simulink model "salirClaseStateFlow"  (R2021b)
settings: Solver=FixedStepAuto  StartTime=0.0  StopTime=inf  RelTol=1e-3  EnableMultiTasking=on
StartFcn:
  | dg = 0.2
model workspace (MAT data in the model file):
  dg = 0.2
settings Model: ExtModeTrigDuration=2  Creator=Mauri  LastModifiedBy=Mauri
settings OptimizationCC: EnhancedBackFolding=on  PassReuseOutputArgsAs=Individual arguments  ZeroExternalMemoryAtStartup=off  ZeroInternalMemoryAtStartup=off  MaxStackSize=64  OptimizeBlockOrder=speed  DifferentSizesBufferReuse=on  OptimizationCustomize=off  EfficientTunableParamExpr=on
settings DebuggingCC: ParameterTunabilityLossMsg=error
settings HardwareCC: ProdBitPerInt=16  ProdBitPerPointer=16  ProdBitPerSizeT=16  ProdBitPerPtrDiffT=16  ProdLargestAtomicFloat=None  ProdWordSize=8  ProdHWDeviceType=Atmel->AVR  UseEmbeddedCoderFeatures=off  UseSimulinkCoderFeatures=off
settings SFSimCC: MATLABDynamicMemAlloc=off
settings RTWCC: Description=Embedded Coder  SystemTargetFile=ert.tlc  HardwareBoard=Arduino Mega 2560  TemplateMakefile=ert_default_tmf  Toolchain=Arduino AVR  BuildConfiguration=Faster Runs
settings CodeAppCC: ForceParamTrailComments=on  IgnoreCustomStorageClasses=off  OperatorAnnotations=on  SimulinkDataObjDesc=on  SFDataObjDesc=on  InsertBlockDesc=on
settings ERTTargetCC: SupportContinuousTime=on  SupportNonInlinedSFcns=on  SupportVariableSizeSignals=on  ExtModeTransport=3  ExtModeStaticAlloc=on  ExtModeStaticAllocSize=2048  ExtModeMexFile=ext_xcp  ExtModeIntrfLevel=Level2 - Open

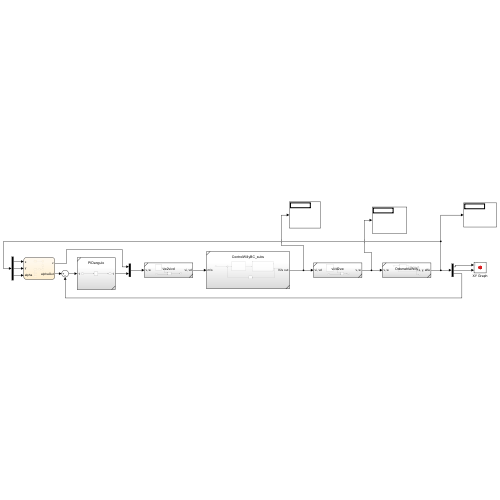
[thumbnail: Simulink's stored preview of the top-level diagram]
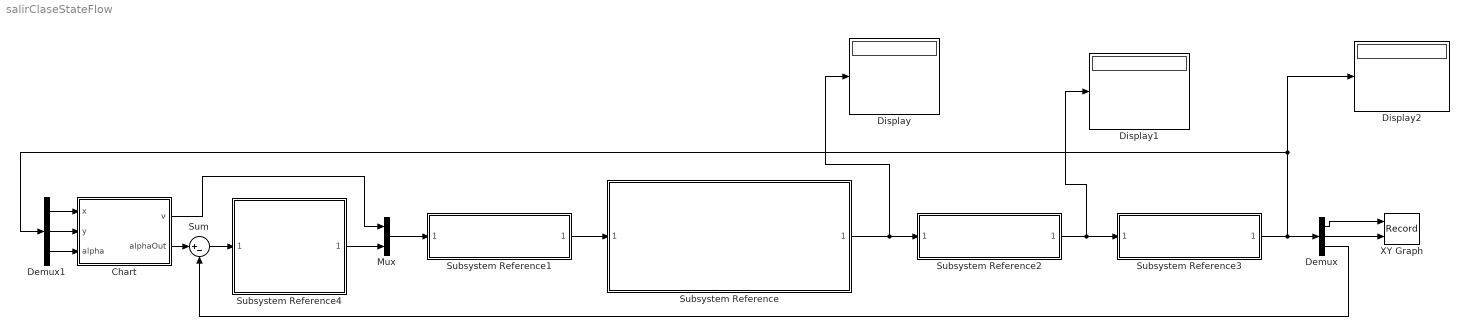
== system salirClaseStateFlow ==
  Chart : Stateflow chart  TreatAsAtomicUnit=on
  Demux : Demux  Outputs=3
  Demux1 : Demux  Outputs=3
  Display : Display
  Display1 : Display
  Display2 : Display
  Mux : Mux  Inputs=2
  Subsystem Reference : Subsystem  ReferencedSubsystem=ControlWillyBC_subs
  Subsystem Reference1 : Subsystem  ReferencedSubsystem=vw2vivd
  Subsystem Reference2 : Subsystem  ReferencedSubsystem=vivd2vw
  Subsystem Reference3 : Subsystem  ReferencedSubsystem=OdometriaWilly
  Subsystem Reference4 : Subsystem  ReferencedSubsystem=PIDangulo
  Sum : Sum  Inputs=|+-
  XY Graph : Record  FileSettingsInternal="{\"entries\":[{\"content\":{\"excelSettings\":{\"content\":{},\"type\":\"Streamout.ExcelSettings\"}},\"type\":\"Streamout.FileSettingStorage\",\"uuid\":\"7011ec7d-dbb6-488a-81e1-d2fabea6677b\"}],\"packageUris\":[\"http://schema.mathworks.com/mf0/streamout_blocks/R2020a\"],\"version\":\"1.0\"}"  Layout=[1 1]  SignalsInternal="{\"entries\":[{\"content\":{\"signals\":[{\"content\":{\"blockPath\":[\"untitled/XY Graph\"],\"channel\":[],\"dimensions\":[1],\"domain\":\"untitled/XY Graph\",\"lineColor\":\"#a2142f\",\"plots\":[1],\"port\":1,\"sid\":[\"\"],\"signalID\":384,\"signalName\":\"Demux:1\"},\"type\":\"RecordBlkView.Signal\",\"uuid\":\"986cc245-256b-4e2e-a10f-a24d8d5d8406\"},{\"content\":{\"blockPath\":[\"untitled/XY Graph\"],\"channel\":[],\"dimensions\":[1],\"domain\":\"untitled/XY Graph\",\"lineColor\":\"#139fff\",\"plots\":[1],\"port\":2,\"sid\":[\"\"],\"signalID\":388,\"signalName\":\"Demux:2\"},\"type\":\"RecordBlkView.Signal\",\"uuid\":\"00b10eef-89a5-46fa-896d-a532f4bbdb0b\"}]},\"type\":\"RecordBlkView.InputSignals\",\"uuid\":\"6d0fa93a-a71f-40d7-b94e-043a5072c355\"}],\"packageUris\":[\"http://schema.mathworks.com/mf0/streamout_blocks/R2020a\"],\"version\":\"1.0\"}"  VisualizationBindings="{\"xyplotplugin\":{\"info\":[{\"series\":[{\"bindingParametersList\":[{\"parameter\":\"X-Axis\",\"signalID\":384,\"signalName\":\"Demux:1\"},{\"parameter\":\"Y-Axis\",\"signalID\":388,\"signalName\":\"Demux:2\"}],\"seriesID\":35200}],\"subplotID\":1}]}}"  CompatibilityTag=XY
  wires:
  Subsystem Reference4/1 -> Mux/2
  Demux/1 -> XY Graph/1
  Mux/1 -> Subsystem Reference1/1
  Demux/2 -> XY Graph/2
  Subsystem Reference3/1 -> Display2/1, Demux1/1, Demux/1
  Subsystem Reference/1 -> Display/1, Subsystem Reference2/1
  Subsystem Reference1/1 -> Subsystem Reference/1
  Subsystem Reference2/1 -> Display1/1, Subsystem Reference3/1
  Chart/1(v) -> Mux/1
  Demux1/1 -> Chart/1(x)
  Demux1/2 -> Chart/2(y)
  Demux1/3 -> Chart/3(alpha)
  Chart/2(alphaOut) -> Sum/1
  Sum/1 -> Subsystem Reference4/1
  Demux/3 -> Sum/2

== stateflow chart salirClaseStateFlow/Chart ==
  state recto1
    entry:
    v = 0.3;
    alphaOut = 0;
  state giro_derecha1
    entry:
    v = 0;
    alphaOut = pi/2;
  state recto2
    entry:
    v = 0.5;
  state giroizquierda
    entry:
    v = 0;
    alphaOut = pi/2;
  state recto3
    entry:
    v = 0.3;
  state giro_derecha2
    entry:
    v = 0;
    alphaOut = pi;
  state recto4
    entry:
    v = 0.3;
  state Stop_
    entry:
    v = 0;
  (default) -> recto1
  recto1 -> giro_derecha1 : [x >= 3.29 ]
  giro_derecha1 -> recto2 : [alpha >= pi/2 ]
  recto2 -> giro_derecha2 : [y >= 11.52]
  giro_derecha2 -> recto3 : [alpha >= pi ]
  recto3 -> giroizquierda : [x <= 2.88]
  giroizquierda -> recto4 : [alpha <= pi/2 + 0.0001]
  recto4 -> Stop_ : [y >= 16.44]
  data: v output; x input; y input; alpha input; alphaOut output
